simulink model "simulink20marshihi"  (R2024a)
settings: Solver=VariableStepAuto  StartTime=0.0  StopTime=1040  RelTol=1e-3
InitFcn:
  | step_initial = get_param('simulink16marshihi/Échelon', 'Before');
  | set_param('simulink16marshihi/Température initiale', 'Value', step_initial);
  | set_param('simulink16marshihi/Chauffage/po_chauffage', 'Value', step_initial);
  | set_param('simulink16marshihi/Refroidissement/po_refroidissement', 'Value', step_initial);
  | consigne = get_param('simulink16marshihi/Échelon', 'After');
  | consigne = str2double(consigne);
  | step_initial = str2double(step_initial);
  | five_up = consigne + 0.05*abs(consigne-step_initial);
  | five_down = consigne - 0.05*abs(consigne-step_initial);
  | set_param('simulink16marshihi/+5%', 'Value', num2str(five_up));
  | set_param('simulink16marshihi/-5%', 'Value', num2str(five_down));
settings Model: Creator=sabri  LastModifiedBy=micrp

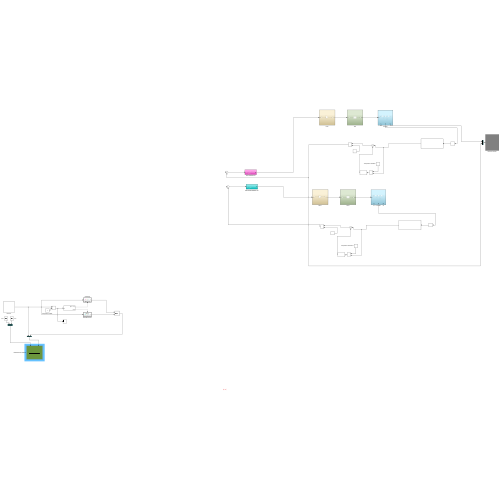
[thumbnail: Simulink's stored preview of the top-level diagram]
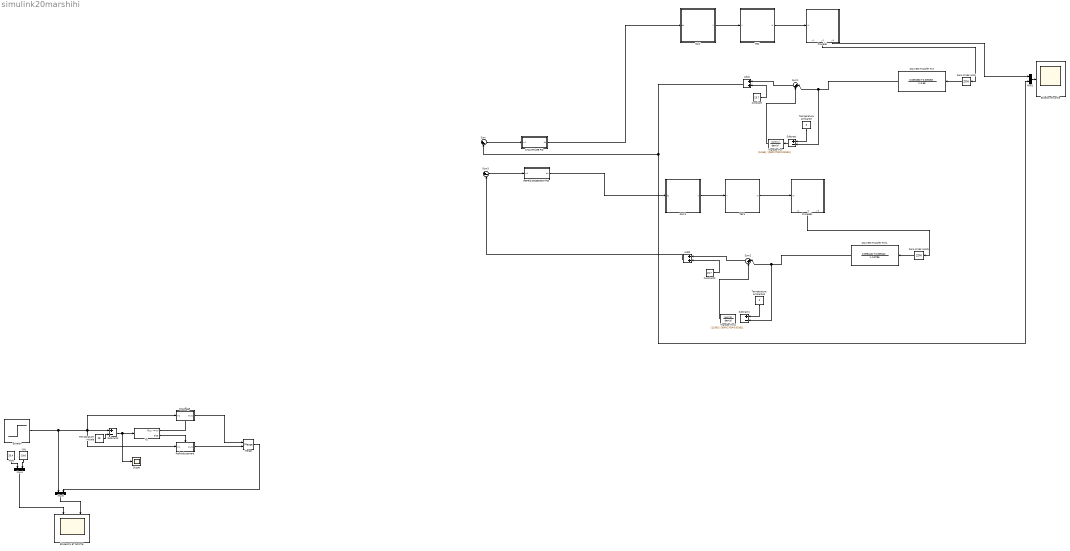
== system simulink20marshihi ==
  " ÉCHELON ET SORTIE" : Scope  NumInputPorts=2
  +5% : Constant  Value=20.4
  -5% : Constant  Value=19.6
  Add1 : Sum
  Add2 : Sum
  CHAUFFAGE PID : Subsystem
  Chauffage : Subsystem  TreatAsAtomicUnit=on
  Constant : Constant  Value=23.7
  Constant3 : Constant  Value=23.7
  DAC : Subsystem
  DAC1 : Subsystem
  Discrete Transfer Fcn : DiscreteTransferFcn  Numerator=[0.009158 0.009158]  Denominator=[1 -0.98]
  Discrete Transfer Fcn1 : DiscreteTransferFcn  Numerator=[0.009442 0.009442]  Denominator=[1 -0.9796]
  If1 : If  IfExpression=u1 >= 0
  Merge : Merge
  Mux1 : Mux  Inputs=2
  Mux4 : Mux  Inputs=2
  Mux5 : Mux  Inputs=2
  Procédé : Subsystem
      settings: PortSchema="{\"entries\":[{\"content\":{\"sides\":[{\"content\":{\"connectorIds\":[\"In1\"]},\"type\":\"ConnectorPlacement.EquallySpacedRectSide\",\"uuid\":\"20a23230-a41b-4fdf-8ae4-039aa17abee7\"},{\"content\":{\"side\":\"RIGHT\"},\"type\":\"ConnectorPlacement.EquallySpacedRectSide\",\"uuid\":\"82e4e468-e0ad-4c9f-b6ff-cc9c1ee7ea9d\"},{\"content\":{\"side\":\"TOP\"},\"type\":\"ConnectorPlacement.EquallySpacedRectSide\",\"uuid\":\"049bc4af-9a9a-43aa-9803-dca862d69d2b\"},{\"content\":{\"connectorIds\":[\"Out1\",\"Out2\",\"Out3\"],\"side\":\"BOTTOM\"},\"type\":\"ConnectorPlacement.EquallySpacedRectSide\",\"uuid\":\"142d2b37-1c32-477b-9e70-4e4bc8b2913e\"}]},\"type\":\"ConnectorPlacement.EquallySpacedConnector\",\"uuid\":\"a0abf580-2deb-4a1c-9cb8-1272669a26fd\"}],\"packageUris\":[\"http://schema.mathworks.com/mf0/Connector/R2020b\"],\"version\":\"1.0\"}"
  Procédé1 : Subsystem
      settings: PortSchema="{\"entries\":[{\"content\":{\"sides\":[{\"content\":{\"connectorIds\":[\"In1\"]},\"type\":\"ConnectorPlacement.EquallySpacedRectSide\",\"uuid\":\"20a23230-a41b-4fdf-8ae4-039aa17abee7\"},{\"content\":{\"side\":\"RIGHT\"},\"type\":\"ConnectorPlacement.EquallySpacedRectSide\",\"uuid\":\"82e4e468-e0ad-4c9f-b6ff-cc9c1ee7ea9d\"},{\"content\":{\"side\":\"TOP\"},\"type\":\"ConnectorPlacement.EquallySpacedRectSide\",\"uuid\":\"049bc4af-9a9a-43aa-9803-dca862d69d2b\"},{\"content\":{\"connectorIds\":[\"Out1\",\"Out2\",\"Out3\"],\"side\":\"BOTTOM\"},\"type\":\"ConnectorPlacement.EquallySpacedRectSide\",\"uuid\":\"142d2b37-1c32-477b-9e70-4e4bc8b2913e\"}]},\"type\":\"ConnectorPlacement.EquallySpacedConnector\",\"uuid\":\"a0abf580-2deb-4a1c-9cb8-1272669a26fd\"}],\"packageUris\":[\"http://schema.mathworks.com/mf0/Connector/R2020b\"],\"version\":\"1.0\"}"
  REFROIDISSEMENT PID : Subsystem
  Refroidissement : Subsystem  TreatAsAtomicUnit=on
  Scope : Scope
  Subtract : Sum  Inputs=+-
  Subtract1 : Sum  Inputs=+-
  Subtract2 : Sum  Inputs=+-
  Sum : Sum  Inputs=|+-
  Sum1 : Sum  Inputs=|++
  Sum2 : Sum  Inputs=|++
  Sum3 : Sum  Inputs=|+-
  TEC : Subsystem
  TEC1 : Subsystem
  Température ambiante : Constant  Value=0
  Température ambiante1 : Constant  Value=0
  Température initiale : Constant  Value=28
  Transfer Fcn : TransferFcn  Numerator=[13.65]  Denominator=[900*2700*0.00161]
  Transfer Fcn1 : TransferFcn  Numerator=[13.65]  Denominator=[900*2700*0.00161]
  Zero-Order Hold : ZeroOrderHold  SampleTime=0.5
  Zero-Order Hold1 : ZeroOrderHold  SampleTime=0.5
  Échelon : Step  Time=0  Before=28  After=20  SampleTime=0
  Échelon et sortie : Scope
  wires:
  Échelon/1 -> Chauffage/1(In1), Subtract2/1, Refroidissement/1(In1), Mux5/1
  ? -> ?
  Température initiale/1 -> Subtract2/2
  +5%/1 -> Mux4/1
  -5%/1 -> Mux4/2
  If1/1 -> Chauffage/Action
  If1/2 -> Refroidissement/Action
  TEC1/1(W) -> Procédé1/1(W)
  DAC1/1(V) -> TEC1/1(V)
  Procédé1/2(y2) -> Zero-Order Hold1/1
  Température ambiante1/1 -> Subtract1/1
  Sum/1 -> CHAUFFAGE PID/1(In1)
  Sum2/1 -> Add2/1
  Add2/1 -> Sum3/2
  Sum3/1 -> REFROIDISSEMENT PID/1(In1)
  REFROIDISSEMENT PID/1(dc) -> DAC1/1(dc)
  Transfer Fcn1/1 -> Sum2/2
  Zero-Order Hold1/1 -> Discrete Transfer Fcn1/1
  Add1/1 -> Sum/2, Mux1/2
  Procédé/2(y2) -> Zero-Order Hold/1
  Zero-Order Hold/1 -> Discrete Transfer Fcn/1
  Subtract/1 -> Transfer Fcn/1
  Constant/1 -> Add1/2
  Discrete Transfer Fcn1/1 -> Sum2/1, Subtract1/2
  TEC/1(W) -> Procédé/1(W)
  CHAUFFAGE PID/1(dc) -> DAC/1(dc)
  Discrete Transfer Fcn/1 -> Sum1/1, Subtract/2
  Transfer Fcn/1 -> Sum1/2
  DAC/1(V) -> TEC/1(V)
  Sum1/1 -> Add1/1
  Constant3/1 -> Add2/2
  Procédé/3(y3) -> Mux1/1
  Température ambiante/1 -> Subtract/1
  Mux1/1 -> Échelon et sortie/1
  Chauffage/1(Out1) -> Merge/1
  Refroidissement/1(Out1) -> Merge/2
  Merge/1 -> Mux5/2
  Subtract2/1 -> Scope/1, If1/1
  Mux5/1 -> " ÉCHELON ET SORTIE"/2
  Mux4/1 -> " ÉCHELON ET SORTIE"/1

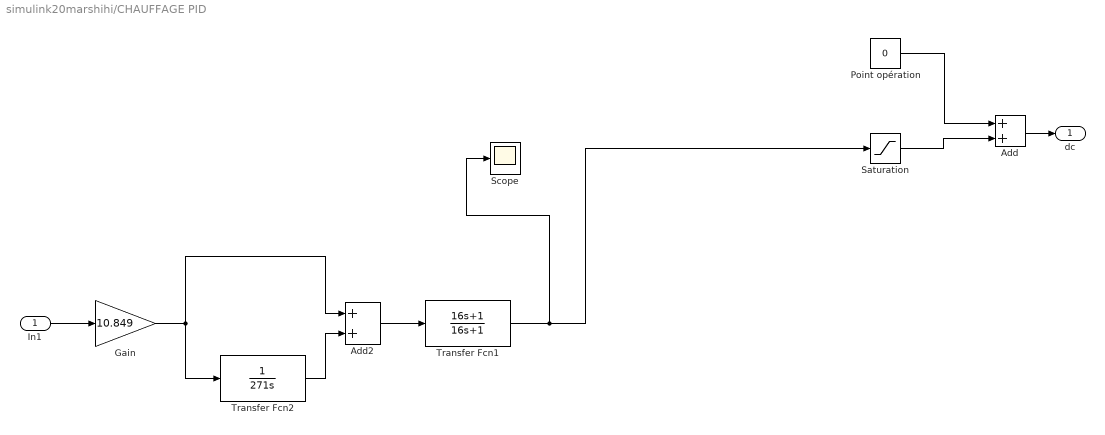
== system simulink20marshihi/CHAUFFAGE PID ==
  In1 : Inport
  Add : Sum
  Add2 : Sum
  Gain : Gain  Gain=10.849
  Point opération : Constant  Value=0
  Saturation : Saturate  UpperLimit=255  LowerLimit=-255
  Scope : Scope
  Transfer Fcn1 : TransferFcn  Numerator=[16 1]  Denominator=[16 1]
  Transfer Fcn2 : TransferFcn  Denominator=[271 0]
  dc : Outport
  wires:
  Add2/1 -> Transfer Fcn1/1
  Saturation/1 -> Add/2
  Point opération/1 -> Add/1
  Transfer Fcn1/1 -> Scope/1, Saturation/1
  Gain/1 -> Transfer Fcn2/1, Add2/1
  Transfer Fcn2/1 -> Add2/2
  In1/1 -> Gain/1
  Add/1 -> dc/1

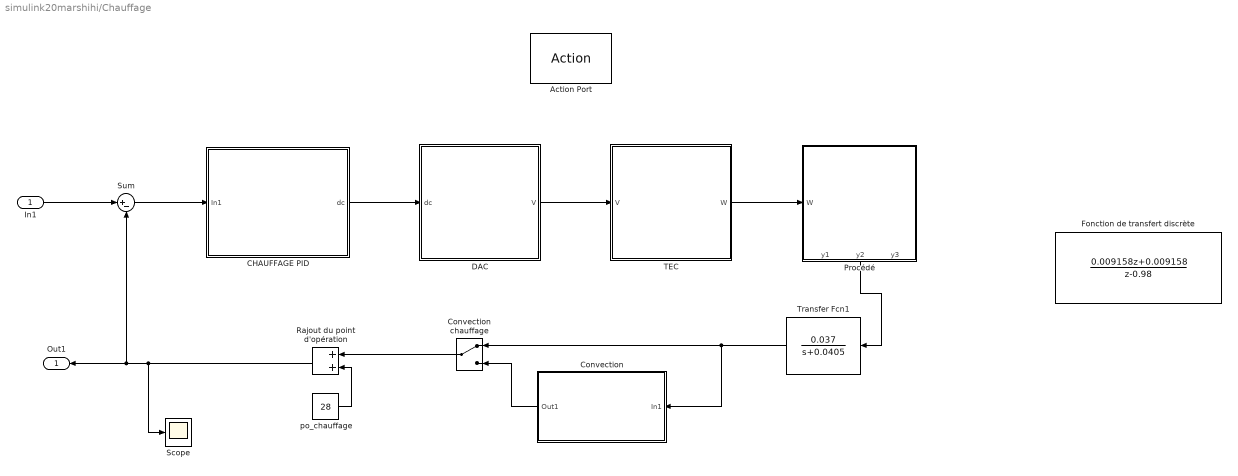
== system simulink20marshihi/Chauffage ==
  In1 : Inport
  Action Port : ActionPort  ActionPortLabel=if(u1 >= 0)
  CHAUFFAGE PID : Subsystem
  Convection : Subsystem
  Convection chauffage : ManualSwitch
  DAC : Subsystem
  Fonction de transfert discrète : DiscreteTransferFcn  Numerator=[0.009158 0.009158]  Denominator=[1 -0.98]
  Procédé : Subsystem
      settings: PortSchema="{\"entries\":[{\"content\":{\"sides\":[{\"content\":{\"connectorIds\":[\"In1\"]},\"type\":\"ConnectorPlacement.EquallySpacedRectSide\",\"uuid\":\"20a23230-a41b-4fdf-8ae4-039aa17abee7\"},{\"content\":{\"side\":\"RIGHT\"},\"type\":\"ConnectorPlacement.EquallySpacedRectSide\",\"uuid\":\"82e4e468-e0ad-4c9f-b6ff-cc9c1ee7ea9d\"},{\"content\":{\"side\":\"TOP\"},\"type\":\"ConnectorPlacement.EquallySpacedRectSide\",\"uuid\":\"049bc4af-9a9a-43aa-9803-dca862d69d2b\"},{\"content\":{\"connectorIds\":[\"Out1\",\"Out2\",\"Out3\"],\"side\":\"BOTTOM\"},\"type\":\"ConnectorPlacement.EquallySpacedRectSide\",\"uuid\":\"142d2b37-1c32-477b-9e70-4e4bc8b2913e\"}]},\"type\":\"ConnectorPlacement.EquallySpacedConnector\",\"uuid\":\"a0abf580-2deb-4a1c-9cb8-1272669a26fd\"}],\"packageUris\":[\"http://schema.mathworks.com/mf0/Connector/R2020b\"],\"version\":\"1.0\"}"
  Rajout du point d'opération : Sum
  Scope : Scope
  Sum : Sum  Inputs=|+-
  TEC : Subsystem
  Transfer Fcn1 : TransferFcn  Numerator=[0.037]  Denominator=[1 0.0405]
  po_chauffage : Constant  Value=28
  Out1 : Outport
  wires:
  Sum/1 -> CHAUFFAGE PID/1(In1)
  In1/1 -> Sum/1
  Rajout du point d'opération/1 -> Scope/1, Out1/1, Sum/2
  TEC/1(W) -> Procédé/1(W)
  CHAUFFAGE PID/1(dc) -> DAC/1(dc)
  DAC/1(V) -> TEC/1(V)
  po_chauffage/1 -> Rajout du point d'opération/2
  Procédé/2(y2) -> Transfer Fcn1/1
  Convection chauffage/1 -> Rajout du point d'opération/1
  Transfer Fcn1/1 -> Convection/1(In1), Convection chauffage/1
  Convection/1(Out1) -> Convection chauffage/2

== system simulink20marshihi/DAC ==
  dc : Inport
  Slope : Gain  Gain=0.079
  V : Outport
  wires:
  dc/1 -> Slope/1
  Slope/1 -> V/1

== system simulink20marshihi/DAC1 ==
  dc : Inport
  Slope : Gain  Gain=0.079
  V : Outport
  wires:
  dc/1 -> Slope/1
  Slope/1 -> V/1

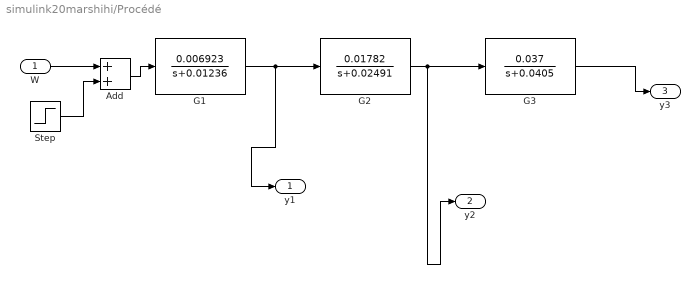
== system simulink20marshihi/Procédé ==
  W : Inport
  Add : Sum
  G1 : TransferFcn  Numerator=[0.006923]  Denominator=[1 0.01236]
  G2 : TransferFcn  Numerator=[0.01782]  Denominator=[1 0.02491]
  G3 : TransferFcn  Numerator=[0.037]  Denominator=[1 0.0405]
  Step : Step  Time=60  After=0  SampleTime=0
  y1 : Outport
  y2 : Outport  Port=2
  y3 : Outport  Port=3
  wires:
  G1/1 -> y1/1, G2/1
  Add/1 -> G1/1
  W/1 -> Add/1
  Step/1 -> Add/2
  G2/1 -> G3/1, y2/1
  G3/1 -> y3/1

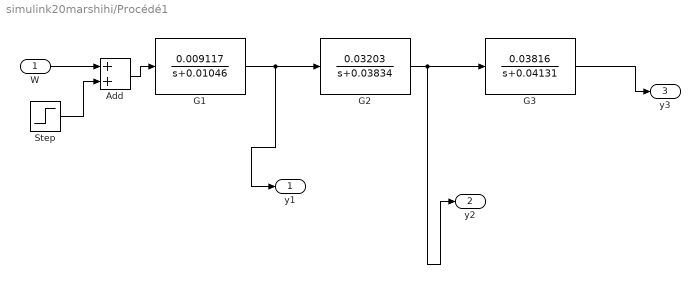
== system simulink20marshihi/Procédé1 ==
  W : Inport
  Add : Sum
  G1 : TransferFcn  Numerator=[0.009117]  Denominator=[1 0.01046]
  G2 : TransferFcn  Numerator=[0.03203]  Denominator=[1 0.03834]
  G3 : TransferFcn  Numerator=[0.03816]  Denominator=[1 0.04131]
  Step : Step  Time=60  After=0  SampleTime=0
  y1 : Outport
  y2 : Outport  Port=2
  y3 : Outport  Port=3
  wires:
  G1/1 -> y1/1, G2/1
  Add/1 -> G1/1
  W/1 -> Add/1
  Step/1 -> Add/2
  G2/1 -> G3/1, y2/1
  G3/1 -> y3/1

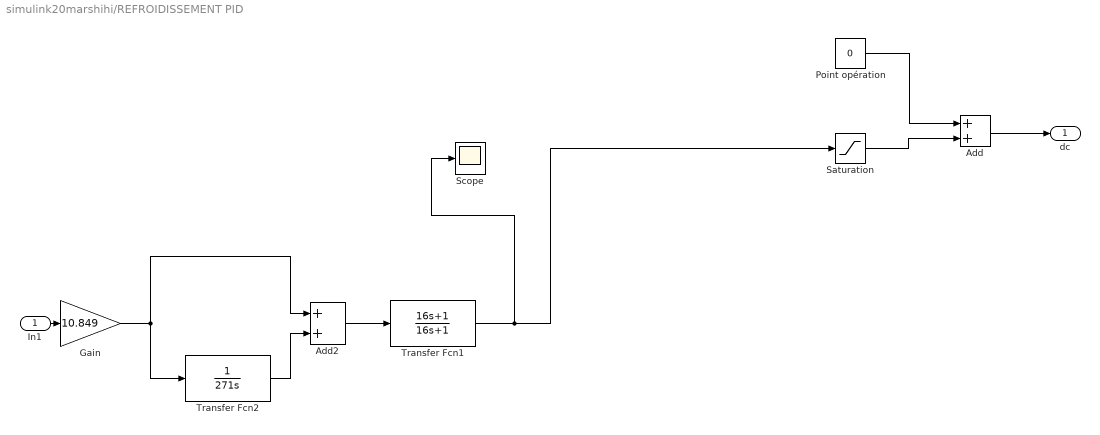
== system simulink20marshihi/REFROIDISSEMENT PID ==
  In1 : Inport
  Add : Sum
  Add2 : Sum
  Gain : Gain  Gain=10.849
  Point opération : Constant  Value=0
  Saturation : Saturate  UpperLimit=255  LowerLimit=-255
  Scope : Scope
  Transfer Fcn1 : TransferFcn  Numerator=[16 1]  Denominator=[16 1]
  Transfer Fcn2 : TransferFcn  Denominator=[271 0]
  dc : Outport
  wires:
  Add2/1 -> Transfer Fcn1/1
  Saturation/1 -> Add/2
  Point opération/1 -> Add/1
  Transfer Fcn1/1 -> Scope/1, Saturation/1
  Gain/1 -> Transfer Fcn2/1, Add2/1
  Transfer Fcn2/1 -> Add2/2
  In1/1 -> Gain/1
  Add/1 -> dc/1

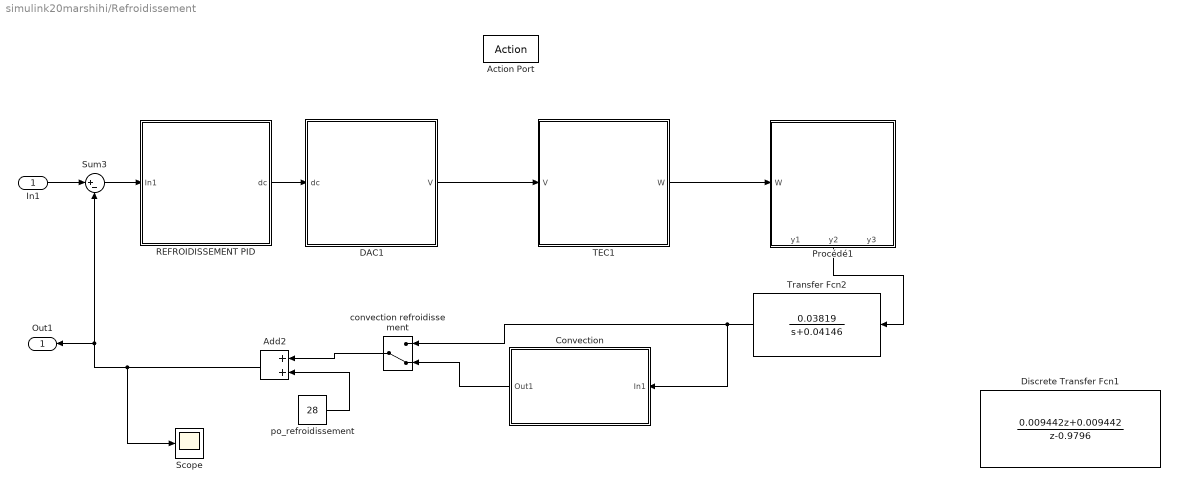
== system simulink20marshihi/Refroidissement ==
  In1 : Inport
  Action Port : ActionPort  ActionPortLabel=else
  Add2 : Sum
  Convection : Subsystem
  DAC1 : Subsystem
  Discrete Transfer Fcn1 : DiscreteTransferFcn  Numerator=[0.009442 0.009442]  Denominator=[1 -0.9796]
  Procédé1 : Subsystem
      settings: PortSchema="{\"entries\":[{\"content\":{\"sides\":[{\"content\":{\"connectorIds\":[\"In1\"]},\"type\":\"ConnectorPlacement.EquallySpacedRectSide\",\"uuid\":\"20a23230-a41b-4fdf-8ae4-039aa17abee7\"},{\"content\":{\"side\":\"RIGHT\"},\"type\":\"ConnectorPlacement.EquallySpacedRectSide\",\"uuid\":\"82e4e468-e0ad-4c9f-b6ff-cc9c1ee7ea9d\"},{\"content\":{\"side\":\"TOP\"},\"type\":\"ConnectorPlacement.EquallySpacedRectSide\",\"uuid\":\"049bc4af-9a9a-43aa-9803-dca862d69d2b\"},{\"content\":{\"connectorIds\":[\"Out1\",\"Out2\",\"Out3\"],\"side\":\"BOTTOM\"},\"type\":\"ConnectorPlacement.EquallySpacedRectSide\",\"uuid\":\"142d2b37-1c32-477b-9e70-4e4bc8b2913e\"}]},\"type\":\"ConnectorPlacement.EquallySpacedConnector\",\"uuid\":\"a0abf580-2deb-4a1c-9cb8-1272669a26fd\"}],\"packageUris\":[\"http://schema.mathworks.com/mf0/Connector/R2020b\"],\"version\":\"1.0\"}"
  REFROIDISSEMENT PID : Subsystem
  Scope : Scope
  Sum3 : Sum  Inputs=|+-
  TEC1 : Subsystem
  Transfer Fcn2 : TransferFcn  Numerator=[0.03819]  Denominator=[1 0.04146]
  convection refroidissement : ManualSwitch  CurrentSetting=0
  po_refroidissement : Constant  Value=28
  Out1 : Outport
  wires:
  TEC1/1(W) -> Procédé1/1(W)
  DAC1/1(V) -> TEC1/1(V)
  Procédé1/2(y2) -> Transfer Fcn2/1
  po_refroidissement/1 -> Add2/2
  Add2/1 -> Scope/1, Out1/1, Sum3/2
  Sum3/1 -> REFROIDISSEMENT PID/1(In1)
  REFROIDISSEMENT PID/1(dc) -> DAC1/1(dc)
  In1/1 -> Sum3/1
  Transfer Fcn2/1 -> Convection/1(In1), convection refroidissement/1
  convection refroidissement/1 -> Add2/1
  Convection/1(Out1) -> convection refroidissement/2

== system simulink20marshihi/TEC ==
  V : Inport
  MATLAB Function : MATLAB Function  TreatAsAtomicUnit=on
  W : Outport
  wires:
  V/1 -> MATLAB Function/1(u)
  MATLAB Function/1(y) -> W/1

== system simulink20marshihi/TEC1 ==
  V : Inport
  MATLAB Function : MATLAB Function  TreatAsAtomicUnit=on
  W : Outport
  wires:
  V/1 -> MATLAB Function/1(u)
  MATLAB Function/1(y) -> W/1

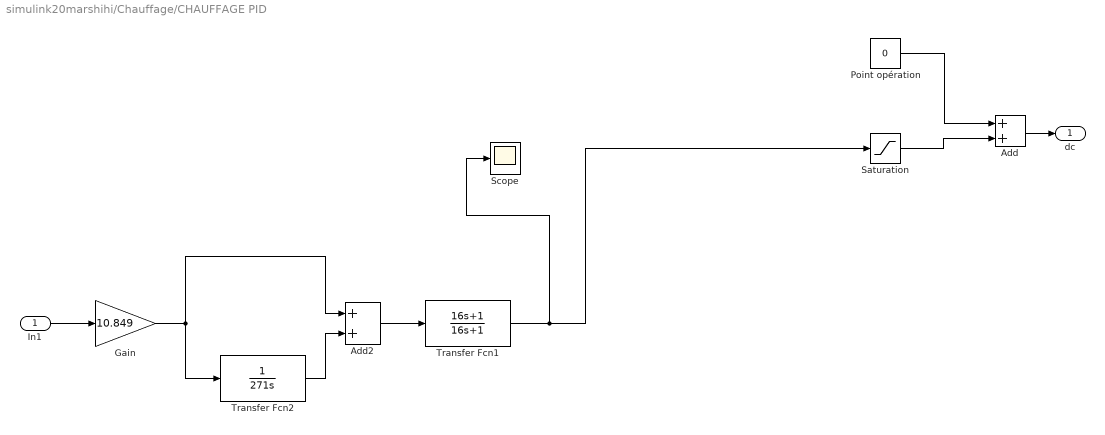
== system simulink20marshihi/Chauffage/CHAUFFAGE PID ==
  In1 : Inport
  Add : Sum
  Add2 : Sum
  Gain : Gain  Gain=10.849
  Point opération : Constant  Value=0
  Saturation : Saturate  UpperLimit=255  LowerLimit=-255
  Scope : Scope
  Transfer Fcn1 : TransferFcn  Numerator=[16 1]  Denominator=[16 1]
  Transfer Fcn2 : TransferFcn  Denominator=[271 0]
  dc : Outport
  wires:
  Add2/1 -> Transfer Fcn1/1
  Saturation/1 -> Add/2
  Point opération/1 -> Add/1
  Transfer Fcn1/1 -> Scope/1, Saturation/1
  Gain/1 -> Transfer Fcn2/1, Add2/1
  Transfer Fcn2/1 -> Add2/2
  In1/1 -> Gain/1
  Add/1 -> dc/1

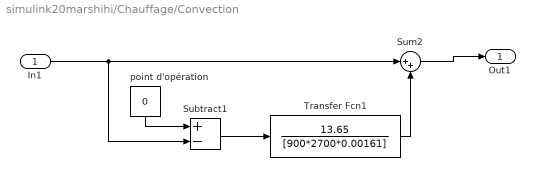
== system simulink20marshihi/Chauffage/Convection ==
  In1 : Inport
  Subtract1 : Sum  Inputs=+-
  Sum2 : Sum  Inputs=|++
  Transfer Fcn1 : TransferFcn  Numerator=[13.65]  Denominator=[900*2700*0.00161]
  point d'opération : Constant  Value=0
  Out1 : Outport
  wires:
  Sum2/1 -> Out1/1
  In1/1 -> Subtract1/2, Sum2/1
  point d'opération/1 -> Subtract1/1
  Subtract1/1 -> Transfer Fcn1/1
  Transfer Fcn1/1 -> Sum2/2

== system simulink20marshihi/Chauffage/DAC ==
  dc : Inport
  Slope : Gain  Gain=0.079
  V : Outport
  wires:
  dc/1 -> Slope/1
  Slope/1 -> V/1

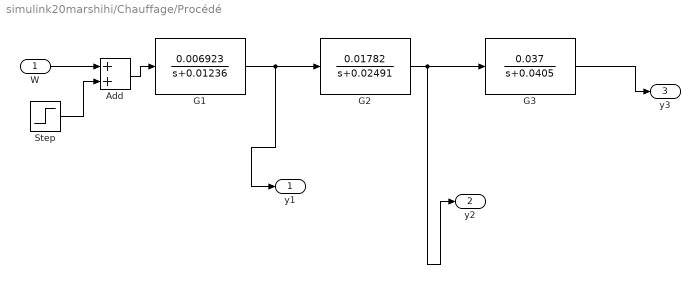
== system simulink20marshihi/Chauffage/Procédé ==
  W : Inport
  Add : Sum
  G1 : TransferFcn  Numerator=[0.006923]  Denominator=[1 0.01236]
  G2 : TransferFcn  Numerator=[0.01782]  Denominator=[1 0.02491]
  G3 : TransferFcn  Numerator=[0.037]  Denominator=[1 0.0405]
  Step : Step  Time=60  After=0  SampleTime=0
  y1 : Outport
  y2 : Outport  Port=2
  y3 : Outport  Port=3
  wires:
  G1/1 -> y1/1, G2/1
  Add/1 -> G1/1
  W/1 -> Add/1
  Step/1 -> Add/2
  G2/1 -> G3/1, y2/1
  G3/1 -> y3/1

== system simulink20marshihi/Chauffage/TEC ==
  V : Inport
  MATLAB Function : MATLAB Function  TreatAsAtomicUnit=on
  W : Outport
  wires:
  V/1 -> MATLAB Function/1(u)
  MATLAB Function/1(y) -> W/1

== system simulink20marshihi/Refroidissement/Convection ==
  In1 : Inport
  Subtract1 : Sum  Inputs=+-
  Sum2 : Sum  Inputs=|++
  Transfer Fcn1 : TransferFcn  Numerator=[13.65]  Denominator=[900*2700*0.00161]
  point d'opération : Constant  Value=0
  Out1 : Outport
  wires:
  Sum2/1 -> Out1/1
  In1/1 -> Subtract1/2, Sum2/1
  point d'opération/1 -> Subtract1/1
  Subtract1/1 -> Transfer Fcn1/1
  Transfer Fcn1/1 -> Sum2/2

== system simulink20marshihi/Refroidissement/DAC1 ==
  dc : Inport
  Slope : Gain  Gain=0.079
  V : Outport
  wires:
  dc/1 -> Slope/1
  Slope/1 -> V/1

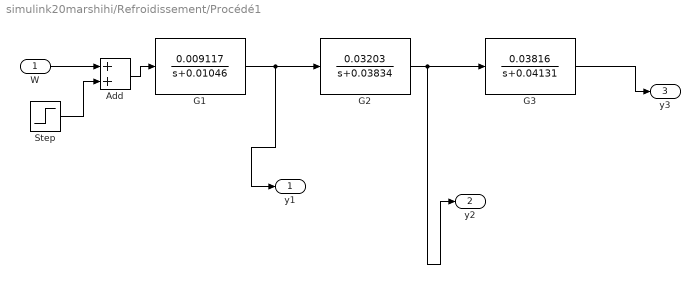
== system simulink20marshihi/Refroidissement/Procédé1 ==
  W : Inport
  Add : Sum
  G1 : TransferFcn  Numerator=[0.009117]  Denominator=[1 0.01046]
  G2 : TransferFcn  Numerator=[0.03203]  Denominator=[1 0.03834]
  G3 : TransferFcn  Numerator=[0.03816]  Denominator=[1 0.04131]
  Step : Step  Time=60  After=0  SampleTime=0
  y1 : Outport
  y2 : Outport  Port=2
  y3 : Outport  Port=3
  wires:
  G1/1 -> y1/1, G2/1
  Add/1 -> G1/1
  W/1 -> Add/1
  Step/1 -> Add/2
  G2/1 -> G3/1, y2/1
  G3/1 -> y3/1

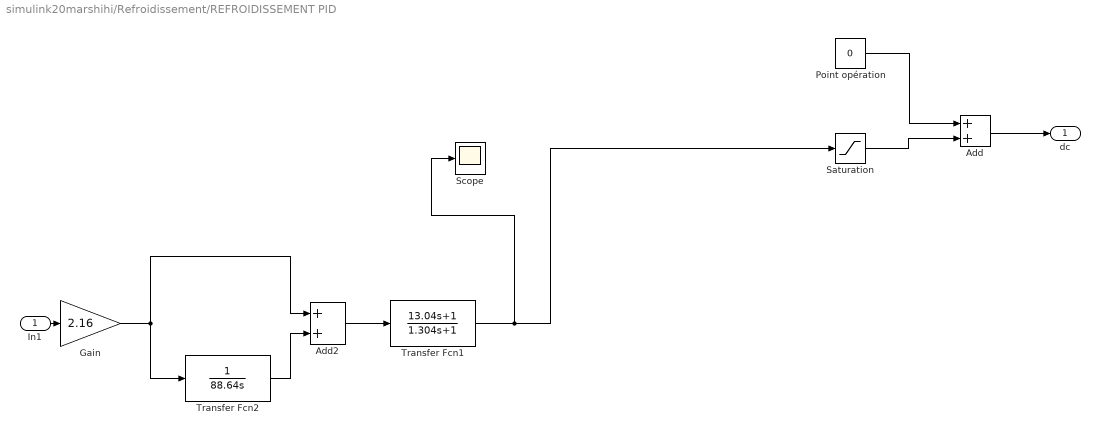
== system simulink20marshihi/Refroidissement/REFROIDISSEMENT PID ==
  In1 : Inport
  Add : Sum
  Add2 : Sum
  Gain : Gain  Gain=2.16
  Point opération : Constant  Value=0
  Saturation : Saturate  UpperLimit=255  LowerLimit=-255
  Scope : Scope
  Transfer Fcn1 : TransferFcn  Numerator=[13.04 1]  Denominator=[1.304 1]
  Transfer Fcn2 : TransferFcn  Denominator=[88.64 0]
  dc : Outport
  wires:
  Add2/1 -> Transfer Fcn1/1
  Saturation/1 -> Add/2
  Point opération/1 -> Add/1
  Transfer Fcn1/1 -> Scope/1, Saturation/1
  Gain/1 -> Transfer Fcn2/1, Add2/1
  Transfer Fcn2/1 -> Add2/2
  In1/1 -> Gain/1
  Add/1 -> dc/1

== system simulink20marshihi/Refroidissement/TEC1 ==
  V : Inport
  MATLAB Function : MATLAB Function  TreatAsAtomicUnit=on
  W : Outport
  wires:
  V/1 -> MATLAB Function/1(u)
  MATLAB Function/1(y) -> W/1

== matlab function simulink20marshihi/TEC1/MATLAB Function ==
  data: u input; y output
function y = fcn(u)
y=6.15*u;

== matlab function simulink20marshihi/TEC/MATLAB Function ==
  data: u input; y output
function y = fcn(u)
y=6.15*u;

== matlab function simulink20marshihi/Chauffage/TEC/MATLAB Function ==
  data: u input; y output
function y = fcn(u)
y=6.15*u;

== matlab function simulink20marshihi/Refroidissement/TEC1/MATLAB Function ==
  data: u input; y output
function y = fcn(u)
y=6.15*u;
